simulink model "stage7"  (Simulink 7.7)
settings: Solver=ode45  StartTime=0.0  StopTime=1  RelTol=1e-3
undefined symbols (not defined in the file): Acid, Lead
libraries: powerlib x9, simulink x2, dsparch4 x1, electricdrivelib x1
settings Model: Creator=Vikas  LastModifiedBy=HASANTH

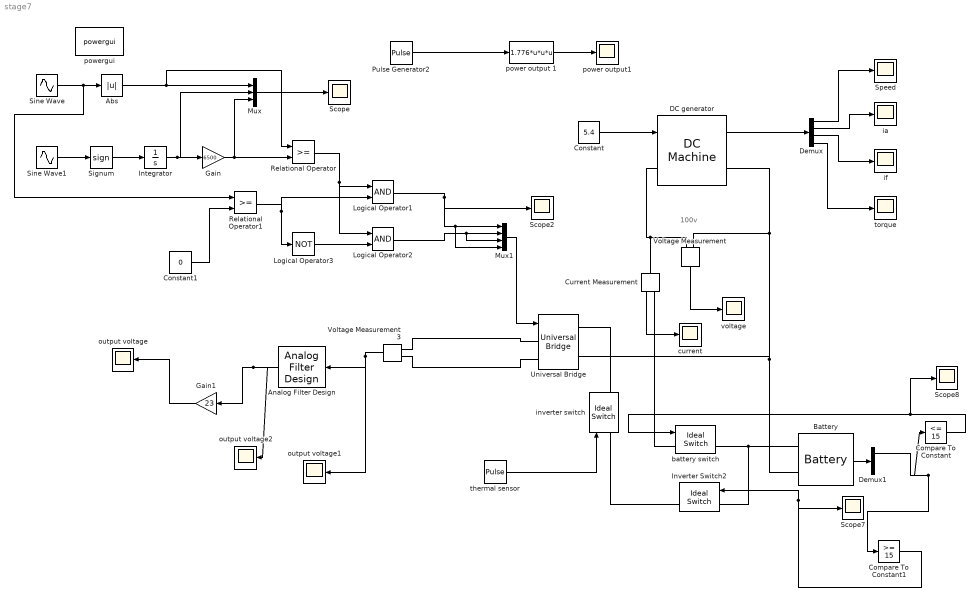
== system stage7 ==
  note: 100v
  Abs : Abs
  Analog Filter Design : dsparch4/Analog Filter Design  method=Butterworth  filttype=Lowpass  N=2  Wlo=30  Whi=80  Rp=2  Rs=40
  Battery : electricdrivelib/Extra Sources/Battery  SystemSampleTime=-1  BatType=Lead-Acid  ShowDetailedParameters=off  NomV=15  NomQ=60  SOC=50  PresetModel=on  MaxQ=62.5  FullV=16.3322  Dis_rate=12  R=0.0025  Normal_OP=18.6167  expZone="[15.2714          0.2]"  Dis_Char=off  current=[6.5 13 32.5]  Units=Time  Batt_Tr=5
  Compare To Constant : simulink/Logic and Bit Operations/Compare To Constant  SystemSampleTime=-1  relop=<=  const=15  LogicOutDataTypeMode=uint8
  Compare To Constant1 : simulink/Logic and Bit Operations/Compare To Constant  SystemSampleTime=-1  relop=>=  const=15  LogicOutDataTypeMode=uint8
  Constant : Constant  Value=5.4
  Constant1 : Constant  Value=0
  Current Measurement : powerlib/Measurements/Current Measurement  SystemSampleTime=-1  PhasorSimulation=off  OutputType=Complex  PSBequivalent=0
  DC generator : powerlib/Machines/DC Machine  SystemSampleTime=-1  PresetModel=No  MechanicalLoad=Speed w  FieldType=Permanent magnet  ShowDetailedParameters=on  RLa="[ 1  0.012]"  RLf="[ 240  120]"  Laf=1.8  MachineConstant=Back-emf constant (V/rpm)  Ke=3  Kt=3.18  J=1  Bm=0  Tf=0  w0=1  Ifinit=1  TsPowergui=0  TsBlock=-1
      settings: AttributesFormatString=\n
  Demux : Demux
  Demux1 : Demux  Outputs=3
  Gain : Gain  Gain=6500
  Gain1 : Gain  Gain=23
  Integrator : Integrator
  Inverter Switch2 : powerlib/Power Electronics/Ideal Switch  SystemSampleTime=-1  Ron=0.001  Lon=0  IC=0  Rs=1e5  Cs=inf  Measurements=on
  Logical Operator1 : Logic  AllPortsSameDT=off  OutDataTypeStr=boolean
  Logical Operator2 : Logic  AllPortsSameDT=off  OutDataTypeStr=boolean
  Logical Operator3 : Logic  Operator=NOT  AllPortsSameDT=off  OutDataTypeStr=boolean
  Mux : Mux  Inputs=3
  Mux1 : Mux
  Pulse Generator2 : DiscretePulseGenerator  PulseType=Time based  Amplitude=3.84  Period=10  PulseWidth=50
  Relational Operator : RelationalOperator  InputSameDT=on
  Relational Operator1 : RelationalOperator  InputSameDT=on
  Scope{,2,7..8} (4 alike) : Scope
      Scope settings: TimeRange=10  YMin=-0.1  YMax=2.1  SaveName=ScopeData5
      Scope2 settings: TimeRange=1  YMin=-0.1  YMax=2.1  SaveName=ScopeData10
      Scope7 settings: TimeRange=0.1  YMin=0.95  YMax=1.05  SaveName=ScopeData7
      Scope8 settings: TimeRange=0.02  YMin=0.95  YMax=1.05  SaveName=ScopeData9
  Signum : Signum
  Sine Wave : Sin  Frequency=2*pi*50  SampleTime=0
  Sine Wave1 : Sin  Frequency=2*pi*3000  SampleTime=0
  Speed : Scope
  Universal Bridge : powerlib/Power Electronics/Universal Bridge  SystemSampleTime=-1  Arms=2  SnubberResistance=1e5  SnubberCapacitance=inf  Device=MOSFET / Diodes  Ron=1e-3  Lon=0  ForwardVoltages="[  0  0  ]"  ForwardVoltage=0  GTOparameters=[ 10e-6 , 20e-6 ]  IGBTparameters=[ 1e-6 , 2e-6 ]  Measurements=None  Measurements_2=None  converterType=Rectifier
  Voltage Measurement : powerlib/Measurements/Voltage Measurement  SystemSampleTime=-1  PhasorSimulation=off  OutputType=Complex  PSBequivalent=0
  Voltage Measurement3 : powerlib/Measurements/Voltage Measurement  SystemSampleTime=-1  PhasorSimulation=off  OutputType=Complex  PSBequivalent=0
  battery switch : powerlib/Power Electronics/Ideal Switch  SystemSampleTime=-1  Ron=0.001  Lon=0  IC=0  Rs=1e5  Cs=inf  Measurements=on
  current : Scope
      settings: TimeRange=0.04  YMin=16.1786  YMax=16.1788  SaveName=ScopeData6
  ia : Scope
      settings: YMin=-0.023  YMax=0
  if : Scope
      settings: SaveName=ScopeData2
  inverter switch : powerlib/Power Electronics/Ideal Switch  SystemSampleTime=-1  Ron=0.001  Lon=0  IC=0  Rs=1e5  Cs=inf  Measurements=on
  output voltage : Scope
      settings: YMin=-3  YMax=3  SaveName=ScopeData8
  output voltage1 : Scope
      settings: YMin=-13.225  YMax=-12.775  SaveName=ScopeData12
  output voltage2 : Scope
      settings: YMin=-13.225  YMax=-12.775  SaveName=ScopeData14
  power output 1 : Fcn  Expr=1.776*u*u*u
  power output1 : Scope
      settings: YMin=265.673  YMax=293.639  SaveName=ScopeData13
  powergui : powerlib/powergui  Priority=1  SystemSampleTime=-1  SimulationMode=Continuous  SampleTime=50e-6  frequency=60  SPID=off  DisableSnubberDevices=off  DisableRonSwitches=off  DisableVfSwitches=off  SwTol=0  Interpol=off  DisplayEquations=off  FunctionMessages=off  frequencyindice=0  Pbase=100e6  ErrMax=1e-4  Iterations=50  UnitsV=kV  UnitsW=MW  echomessages=off  HookPort=off  EnableUseOfTLC=off  x0status=steady  RestoreLinks=no  ResistiveCurrentMeasurement=off  Frange=[0:2:500]  Ylog=off  Xlog=on  ShowGrid=off  save=off  variable=ZData  structure=ScopeData8  ZoomFFT=off  StartTime=0.0  cycles=1  DisplayStyle=1  fundamental=60  FreqAxis=off  MaxFrequency=1000  frequencyindicesteady=1  RmsSteady=1  display=off  Ts=0  methode=off
  thermal sensor : DiscretePulseGenerator  PulseType=Time based  Period=14400  PulseWidth=50
  torque : Scope
      settings: SaveName=ScopeData3
  voltage : Scope
      settings: TimeRange=0.04  YMin=0.0164395  YMax=0.0164505  SaveName=ScopeData4
  wires:
  DC generator/1 -> Demux/1
  Demux/1 -> Speed/1
  Demux/2 -> ia/1
  Demux/3 -> if/1
  Demux/4 -> torque/1
  Voltage Measurement/1 -> voltage/1
  Sine Wave/1 -> Abs/1, Relational Operator1/1
  Abs/1 -> Mux/1, Relational Operator/1
  Mux/1 -> Scope/1
  Sine Wave1/1 -> Signum/1
  Signum/1 -> Integrator/1
  Integrator/1 -> Mux/2, Gain/1
  Logical Operator3/1 -> Logical Operator2/2
  Relational Operator/1 -> Logical Operator1/1, Logical Operator2/1
  Constant1/1 -> Relational Operator1/2
  Relational Operator1/1 -> Logical Operator3/1, Logical Operator1/2
  Mux1/1 -> Universal Bridge/1
  Logical Operator1/1 -> Mux1/1, Mux1/4, Scope2/1
  Logical Operator2/1 -> Mux1/2, Mux1/3
  Battery/1 -> Demux1/1
  Demux1/1 -> Compare To Constant/1, Compare To Constant1/1
  Compare To Constant/1 -> battery switch/1, Scope8/1
  Voltage Measurement3/1 -> output voltage1/1, Analog Filter Design/1
  Current Measurement/1 -> current/1
  Constant/1 -> DC generator/1
  thermal sensor/1 -> inverter switch/1
  Pulse Generator2/1 -> power output 1/1
  power output 1/1 -> power output1/1
  Gain/1 -> Mux/3, Relational Operator/2
  Analog Filter Design/1 -> Gain1/1, output voltage2/1
  Gain1/1 -> output voltage/1
  Compare To Constant1/1 -> Inverter Switch2/1, Scope7/1
  connections:
  Battery/LConn1 -- battery switch/RConn1 -- Inverter Switch2/LConn1
  Current Measurement/LConn1 -- Voltage Measurement/LConn1 -- DC generator/LConn1
  Voltage Measurement/LConn2 -- DC generator/RConn1 -- Universal Bridge/RConn2 -- Battery/LConn2
  Current Measurement/RConn1 -- battery switch/LConn1
  inverter switch/LConn1 -- Inverter Switch2/RConn1
  inverter switch/RConn1 -- Universal Bridge/RConn1
  Universal Bridge/LConn1 -- Voltage Measurement3/LConn1
  Universal Bridge/LConn2 -- Voltage Measurement3/LConn2
